simulink model "extendidoAkermanLenminiscataBernulliSeguimiento"  (R2023a)
settings: Solver=ode4  StartTime=0.0  StopTime=200  FixedStep=0.02  RelTol=1e-3
settings Model: Creator=uriel  LastModifiedBy=uriel

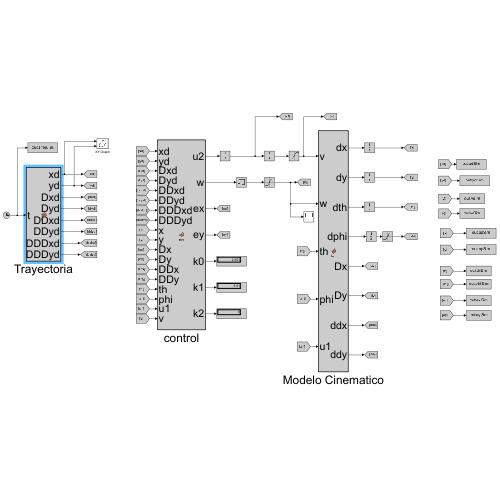
[thumbnail: Simulink's stored preview of the top-level diagram]
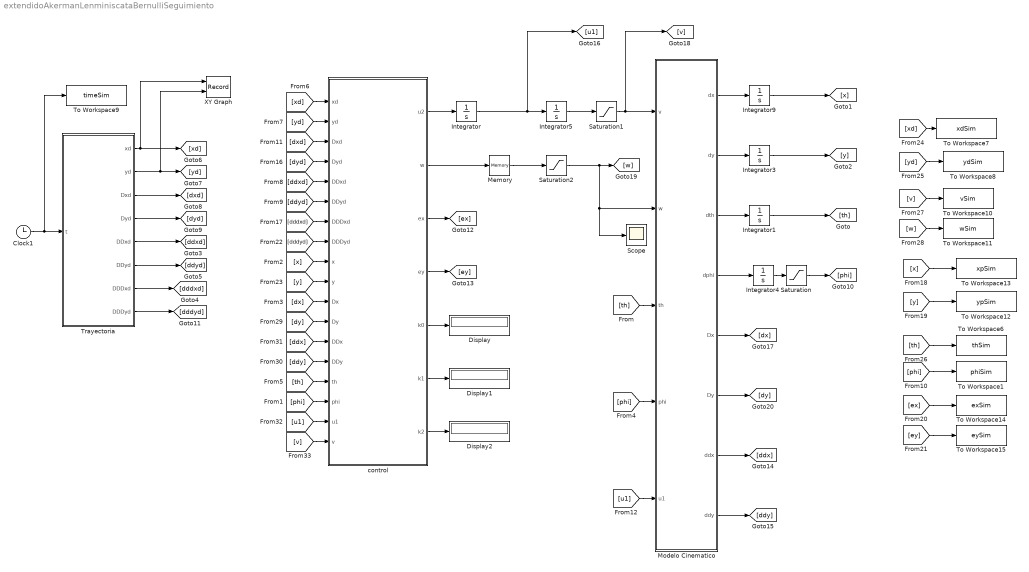
== system extendidoAkermanLenminiscataBernulliSeguimiento ==
  Clock1 : Clock
  Display : Display
  Display1 : Display
  Display2 : Display
  Integrator : Integrator
  Integrator1 : Integrator  InitialCondition=1.66
  Integrator3 : Integrator  InitialCondition=0.0897
  Integrator4 : Integrator
  Integrator5 : Integrator  InitialCondition=0.07
  Integrator9 : Integrator  InitialCondition=2.3473
  Memory : Memory
  Modelo Cinematico : MATLAB Function  TreatAsAtomicUnit=on
  Saturation : Saturate  UpperLimit=0.38  LowerLimit=-0.4
  Saturation1 : Saturate  UpperLimit=1.0  LowerLimit=0.01
  Saturation2 : Saturate  UpperLimit=0.38  LowerLimit=-0.4
  Scope : Scope
  To Workspace1 : ToWorkspace  VariableName=phiSim  SaveFormat=Structure  SampleTime=-1
  To Workspace10 : ToWorkspace  VariableName=vSim  SaveFormat=Structure  SampleTime=-1
  To Workspace11 : ToWorkspace  VariableName=wSim  SaveFormat=Structure  SampleTime=-1
  To Workspace12 : ToWorkspace  VariableName=ypSim  SaveFormat=Structure  SampleTime=-1
  To Workspace13 : ToWorkspace  VariableName=xpSim  SaveFormat=Structure  SampleTime=-1
  To Workspace14 : ToWorkspace  VariableName=exSim  SaveFormat=Structure  SampleTime=-1
  To Workspace15 : ToWorkspace  VariableName=eySim  SaveFormat=Structure  SampleTime=-1
  To Workspace6 : ToWorkspace  VariableName=thSim  SaveFormat=Structure  SampleTime=-1
  To Workspace7 : ToWorkspace  VariableName=xdSim  SaveFormat=Structure  SampleTime=-1
  To Workspace8 : ToWorkspace  VariableName=ydSim  SaveFormat=Structure  SampleTime=-1
  To Workspace9 : ToWorkspace  VariableName=timeSim  SaveFormat=Structure  SampleTime=-1
  Trayectoria : MATLAB Function  TreatAsAtomicUnit=on
  XY Graph : Record  FileSettingsInternal="{\"entries\":[{\"content\":{\"excelSettings\":{\"content\":{},\"type\":\"Streamout.ExcelSettings\"}},\"type\":\"Streamout.FileSettingStorage\",\"uuid\":\"\"}],\"packageUris\":[\"http:\\/\\/schema.mathworks.com\\/mf0\\/streamout_blocks\\/R2020a\"],\"version\":\"1.0\"}"  Layout=[1 1]  SignalsInternal="{\"entries\":[{\"content\":{\"signals\":[{\"content\":{\"blockPath\":[],\"dimensions\":[1],\"domain\":\"\",\"lineColor\":\"#a2142f\",\"plots\":[1],\"port\":1,\"sid\":[\"\"],\"signalID\":718,\"signalName\":\"Trayectoria:1\"},\"type\":\"RecordBlkView.Signal\",\"uuid\":\"\"},{\"content\":{\"blockPath\":[],\"dimensions\":[1],\"domain\":\"\",\"lineColor\":\"#139fff\",\"plots\":[1],\"port\":2,\"sid\":[\"\"],\"signalID\":722,\"signalName\":\"Trayectoria:2\"},\"type\":\"RecordBlkView.Signal\",\"uuid\":\"\"}]},\"type\":\"RecordBlkView.InputSignals\",\"uuid\":\"\"}],\"packageUris\":[\"http:\\/\\/schema.mathworks.com\\/mf0\\/streamout_blocks\\/R2020a\"],\"version\":\"1.0\"}"  VisualizationBindings="{\"xyplotplugin\":{\"info\":[{\"series\":[{\"bindingParametersList\":[{\"parameter\":\"X-Axis\",\"signalID\":718,\"signalName\":\"Trayectoria:1\"},{\"parameter\":\"Y-Axis\",\"signalID\":722,\"signalName\":\"Trayectoria:2\"}],\"seriesID\":37990}],\"subplotID\":1}]}}"  CompatibilityTag=XY
  control : MATLAB Function  TreatAsAtomicUnit=on
  wires:
  [v] -> To Workspace10/1
  [x] -> To Workspace13/1
  Trayectoria/3(Dxd) -> [dxd]
  control/4(ey) -> [ey]
  [th] -> To Workspace6/1
  [xd] -> To Workspace7/1
  [xd] -> control/1(xd)
  [ey] -> To Workspace15/1
  [w] -> To Workspace11/1
  [th] -> Modelo Cinematico/3(th)
  [yd] -> control/2(yd)
  [yd] -> To Workspace8/1
  Trayectoria/2(yd) -> XY Graph/2, [yd]
  control/3(ex) -> [ex]
  Integrator1/1 -> [th]
  Clock1/1 -> To Workspace9/1, Trayectoria/1(t)
  [y] -> To Workspace12/1
  [ex] -> To Workspace14/1
  [phi] -> control/16(phi)
  [phi] -> Modelo Cinematico/4(phi)
  [phi] -> To Workspace1/1
  Saturation/1 -> [phi]
  Integrator4/1 -> Saturation/1
  Trayectoria/8(DDDyd) -> [dddyd]
  [dyd] -> control/4(Dyd)
  [dxd] -> control/3(Dxd)
  [ddxd] -> control/5(DDxd)
  [ddyd] -> control/6(DDyd)
  [dddxd] -> control/7(DDDxd)
  [dddyd] -> control/8(DDDyd)
  [x] -> control/9(x)
  [y] -> control/10(y)
  [dx] -> control/11(Dx)
  [dy] -> control/12(Dy)
  [ddx] -> control/13(DDx)
  [ddy] -> control/14(DDy)
  [th] -> control/15(th)
  [u1] -> control/17(u1)
  [v] -> control/18(v)
  Integrator5/1 -> Saturation1/1
  control/2(w) -> Memory/1
  Memory/1 -> Saturation2/1
  Saturation1/1 -> Modelo Cinematico/1(v), [v]
  Integrator3/1 -> [y]
  [u1] -> Modelo Cinematico/5(u1)
  Modelo Cinematico/3(dth) -> Integrator1/1
  Modelo Cinematico/4(dphi) -> Integrator4/1
  Integrator9/1 -> [x]
  Modelo Cinematico/1(dx) -> Integrator9/1
  Modelo Cinematico/2(dy) -> Integrator3/1
  control/1(u2) -> Integrator/1
  Modelo Cinematico/7(ddx) -> [ddx]
  Modelo Cinematico/8(ddy) -> [ddy]
  Integrator/1 -> [u1], Integrator5/1
  control/5(k0) -> Display/1
  control/6(k1) -> Display1/1
  control/7(k2) -> Display2/1
  Trayectoria/7(DDDxd) -> [dddxd]
  Trayectoria/6(DDyd) -> [ddyd]
  Trayectoria/5(DDxd) -> [ddxd]
  Trayectoria/4(Dyd) -> [dyd]
  Modelo Cinematico/5(Dx) -> [dx]
  Modelo Cinematico/6(Dy) -> [dy]
  Saturation2/1 -> [w], Scope/1, Modelo Cinematico/2(w)
  Trayectoria/1(xd) -> XY Graph/1, [xd]

== matlab function extendidoAkermanLenminiscataBernulliSeguimiento/Modelo Cinematico ==
  data: v input; w input; dx output; th input; dy output; dth output; phi input; dphi output; Dx output; Dy output; u1 input; ddx output; ddy output
function [dx,dy,dth,dphi,Dx,Dy,ddx,ddy]  = fcn(v,w,th,phi,u1)

%%%%%%%%%%%%%% MATRIZ DE DESACOPLAMIENTO %%%%%%%%%%%%%%%%%%%%%55
l=0.26;
%vf=v/cos(phi);
dx=v*cos(th);
dy=v*sin(th);
dth=v*tan(phi)/l;
dphi=w;

Dx = v*cos(th);
Dy = v*sin(th);
ddx=u1*cos(th)-v*v*tan(phi)*sin(th)/l;
ddy=u1*sin(th)+v*v*tan(phi)*cos(th)/l;

== matlab function extendidoAkermanLenminiscataBernulliSeguimiento/Trayectoria ==
  data: xd output; yd output; Dxd output; Dyd output; DDxd output; DDyd output; DDDxd output; t input; DDDyd output
function [xd,yd,Dxd,Dyd,DDxd,DDyd,DDDxd,DDDyd]   = fcn(t)
T=100;
f=1/T;
w=2*pi*f;
a = 2.3;
d = 2.5;

xd = a*cos(w*t)/(1+(sin(w*t)*(sin(w*t))));
Dxd = -a*((w*sin(w*t)/(1+sin(w*t)*sin(w*t)))+2*w*sin(w*t)*cos(w*t)*cos(w*t)/((1+(sin(w*t)*sin(w*t)))*(1+(sin(w*t)*sin(w*t)))));
DDxd = a*(-(w*w*cos(w*t)/(1+sin(w*t)*sin(w*t)))+(6*w*w*sin(w*t)*sin(w*t)*cos(w*t)/((1+sin(w*t)*sin(w*t))*(1+sin(w*t)*sin(w*t))))-(2*w*w*cos(w*t)*cos(w*t)*cos(w*t)/((1+sin(w*t)*sin(w*t))*(1+sin(w*t)*sin(w*t))))+(8*w*w*sin(w*t)*sin(w*t)*cos(w*t)*cos(w*t)*cos(w*t)/((1+sin(w*t)*sin(w*t))*(1+sin(w*t)*sin(w*t))*(1+sin(w*t)*sin(w*t)))));
DDDxd = a*((w*w*w*sin(w*t)/(1+sin(w*t)*sin(w*t)))+(20*w*w*w*sin(w*t)*cos(w*t)*cos(w*t)/((1+sin(w*t)*sin(w*t))*(1+sin(w*t)*sin(w*t))))-(6*w*w*w*sin(w*t)*sin(w*t)*sin(w*t)/((1+sin(w*t)*sin(w*t))*(1+sin(w*t)*sin(w*t))))-(48*w*w*w*sin(w*t)*sin(w*t)*sin(w*t)*cos(w*t)*cos(w*t)/((1+sin(w*t)*sin(w*t))*(1+sin(w*t)*sin(w*t))*(1+sin(w*t)*sin(w*t))))+(24*w*w*w*sin(w*t)*cos(w*t)*cos(w*t)*cos(w*t)*cos(w*t)/((1+sin(w*t)*sin(w*t))*(1+sin(w*t)*sin(w*t))*(1+sin(w*t)*sin(w*t))))-(48*w*w*w*sin(w*t)*sin(w*t)*sin(w*t)*cos(w*t)*cos(w*t)*cos(w*t)*cos(w*t)/((1+sin(w*t)*sin(w*t))*(1+sin(w*t)*sin(w*t))*(1+sin(w*t)*sin(w*t))*(1+sin(w*t)*sin(w*t)))));

yd = d*(sin(w*t)*cos(w*t))/(1+(sin(w*t)*sin(w*t)));
Dyd = d*((w*cos(w*t)*cos(w*t)/(1+sin(w*t)*sin(w*t)))-(w*sin(w*t)*sin(w*t)/(1+sin(w*t)*sin(w*t)))-(2*w*sin(w*t)*sin(w*t)*cos(w*t)*cos(w*t)/((1+sin(w*t)*sin(w*t))*(1+sin(w*t)*sin(w*t)))));
DDyd = d*((-4*w*w*sin(w*t)*cos(w*t)/(1+sin(w*t)*sin(w*t)))-(6*w*w*sin(w*t)*cos(w*t)*cos(w*t)*cos(w*t)/((1+sin(w*t)*sin(w*t))*(1+sin(w*t)*sin(w*t))))+(6*w*w*sin(w*t)*sin(w*t)*sin(w*t)*cos(w*t)/((1+sin(w*t)*sin(w*t))*(1+sin(w*t)*sin(w*t))))+(8*w*w*sin(w*t)*sin(w*t)*sin(w*t)*cos(w*t)*cos(w*t)*cos(w*t)/((1+sin(w*t)*sin(w*t))*(1+sin(w*t)*sin(w*t))*(1+sin(w*t)*sin(w*t)))));
DDDyd = d*((-4*w*w*w*cos(w*t)*cos(w*t)/(1+sin(w*t)*sin(w*t)))+(4*w*w*w*sin(w*t)*sin(w*t)/(1+sin(w*t)*sin(w*t)))+(44*w*w*w*sin(w*t)*sin(w*t)*cos(w*t)*cos(w*t)/((1+sin(w*t)*sin(w*t))*(1+sin(w*t)*sin(w*t))))-(6*w*w*w*cos(w*t)*cos(w*t)*cos(w*t)*cos(w*t)/((1+sin(w*t)*sin(w*t))*(1+sin(w*t)*sin(w*t))))-(6*w*w*w*sin(w*t)*sin(w*t)*sin(w*t)*sin(w*t)/((1+sin(w*t)*sin(w*t))*(1+sin(w*t)*sin(w*t))))+(48*w*w*w*sin(w*t)*sin(w*t)*cos(w*t)*cos(w*t)*cos(w*t)*cos(w*t)/((1+sin(w*t)*sin(w*t))*(1+sin(w*t)*sin(w*t))*(1+sin(w*t)*sin(w*t))))-(48*w*w*w*sin(w*t)*sin(w*t)*sin(w*t)*sin(w*t)*cos(w*t)*cos(w*t)/((1+sin(w*t)*sin(w*t))*(1+sin(w*t)*sin(w*t))*(1+sin(w*t)*sin(w*t))))-(48*w*w*w*sin(w*t)*sin(w*t)*sin(w*t)*sin(w*t)*cos(w*t)*cos(w*t)*cos(w*t)*cos(w*t)/((1+sin(w*t)*sin(w*t))*(1+sin(w*t)*sin(w*t))*(1+sin(w*t)*sin(w*t))*(1+sin(w*t)*sin(w*t)))));

== matlab function extendidoAkermanLenminiscataBernulliSeguimiento/control ==
  data: u2 output; xd input; yd input; Dxd input; Dyd input; DDxd input; DDyd input; DDDxd input; DDDyd input; x input; y input; Dx input; Dy input; DDx input; DDy input; th input; phi input; w output; ex output; ey output; u1 input; v input; k0 output; k1 output; k2 output
function [u2,w,ex,ey,k0,k1,k2 ]   = fcn(xd,yd,Dxd,Dyd,DDxd,DDyd,DDDxd,DDDyd,x,y,Dx,Dy,DDx,DDy,th,phi,u1,v)
l=0.26;
%% Matriz de desacoplamiento
A=[cos(th), -v*v*sin(th)*(1+(tan(phi)*tan(phi)))/l;
   sin(th),  v*v*cos(th)*(1+(tan(phi)*tan(phi)))/l];
%% Matriz de compensanción
B=[-(3*v*u1*sin(th)*tan(phi)/l)-v*v*v*cos(th)*tan(phi)*tan(phi)/(l*l);
   (3*v*u1*cos(th)*tan(phi)/l)-v*v*v*sin(th)*tan(phi)*tan(phi)/(l*l)];
%% Señales de error
ex = x-xd;
ey = y-yd;
Dex = Dx-Dxd;
Dey = Dy-Dyd;
DDex = DDx-DDxd;
DDey = DDy-DDyd;
%% Ganancias de control
z=0.7;
ts=6;
wn=3/(ts*z);

p2=2*z*wn;
p3=wn*wn;
p1=5.0;

k0 = p1*p3;
k1 = p3+p1*p2;
k2 = p1+p2;


% k0 = 0.1;
% k1 = 2;
% k2 = 1;

%z=2;
%ts=12.5;
%wn=4/(ts*z);
%wn=1;
%p2=2*z*wn;
%p3=wn*wn;
%p1=2.5/2;
%k0 = p1*p3;
%%k1 = p3+p1*p2;
%k2 = p1+p2;

%% Control auxiliar
rx=-k0*ex-k1*Dex-k2*DDex+DDDxd;
ry=-k0*ey-k1*Dey-k2*DDey+DDDyd;
r=[rx;ry];

%% Control
U=A\(r-B);
u2 = U(1);
w = U(2);
